simulink library "dspsigattribs"  (Simulink 6.0)
values from neighbouring files (symbols this model uses):
  D = D + B    [rebuffer_delay.m]
libraries: dspsigattribs x2, simulink x1, simulink3 x1
settings Model: RequirementInfo=9  CovMetricSettings=d  Creator=don  LastModifiedBy=mlongfri  ExtModeAutoUpdateStatusClock=off
settings Model: ForwardingTableString=|
  | ||__slOldName__||dspsigattribs/Contiguous
  | Copy||__slNewName__||dspobslib/Contiguous
  | Copy||__slOldName__||dspsigattribs/DSP Fixed-Point
  | Attributes||__slNewName__||dspobslib/DSP Fixed-Point
  | Attributes

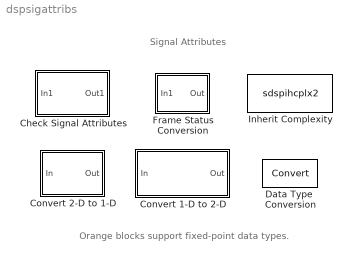
== system dspsigattribs ==
  note: Signal Attributes
  note: Orange blocks support fixed-point data types.
  Check Signal Attributes : Subsystem  mask(Check Signal Attributes){SigAttribCheckMethod=Does not match attributes exactly, Complexity=Ignore, Frame=Ignore, DimsCheckMethod=Ignore, Dimensions=1-D, DatatypeCheckMethod=Ignore, DatatypeGeneral=Boolean, DtypeFloatSpecific=Any floating-point, DtypeFixedSpecific=Any fixed-point, DtypeIntSpecific=Any integer, SampleMode=Ignore}
      mask prompts: SigAttribCheckMethod "Error when input:"; Frame "Frame status:"; DimsCheckMethod "Dimensionality:"; DatatypeCheckMethod "Data type:"; DatatypeGeneral "General data type:"; DtypeFloatSpecific "Specific floating-point:"; DtypeFixedSpecific "Specific fixed-point:"; DtypeIntSpecific "Specific integer:"; SampleMode "Sample mode:"
      mask help: Generate an error when the input signal does or does not match selected attributes exactly.
      settings: CopyFcn=dspfixptcopycallback
      mask Help: web(dspbhelp);
      mask StyleString: popup(Does not match attributes exactly|Matches attributes exactly),popup(Ignore|Real|Complex),popup(Ignore|Frame-based|Sample-based),popup(Ignore|Is...|Is not...),popup(1-D|2-D|Scalar (1-D or 2-D)|Vector (1-D or 2-D)|Vector (1-D or 2-D) or scalar|Row vector (2-D)|Row vector (2-D) or scalar|Column vector (2-D)|Column vector (2-D) or scalar|Full matrix (2-D)|Square matrix (2-D)),popup(Ignore|Is...|Is not...),popup(Boolean|Floating-point|Fixed-point|Integer),popup(Any floating-point|Double precision|Single precision),popup(Any fixed-point|Signed fixed-point|Unsigned fixed-point),popup(Any integer|Signed integer|Unsigned integer|int8|int16|int32|uint8|uint16|uint32),popup(Ignore|Discrete|Continuous)
      mask CallbackString: |||dspblkchksigattrbs||dspblkchksigattrbs|dspblkchksigattrbs|||dspblkchksigattrbs|
      mask Display: disp('Check Signal\n Attributes');
  Convert 1-D to 2-D : Subsystem  mask(Convert 1-D to 2-D){M=1, N=1, frameBasedOut=off}
      mask prompts: M "Number of output rows:"; N "Number of output columns:"; frameBasedOut "Frame-based output"
      mask help: Output a (2-D) matrix signal.
      mask init:
      | dspblkcnvrt1d2d;
      settings: CopyFcn=dspfixptcopycallback
      mask Help: web(dspbhelp);
      mask Display: disp('reshape(U,M,N)')
  Convert 2-D to 1-D : Subsystem
      settings: CopyFcn=dspfixptcopycallback
      mask Type: Convert 2-D to 1-D
      mask Description: Output a (1-D) vector signal.
      mask Help: web(dspbhelp);
      mask Display: disp('U( : )')
  Data Type  Conversion : DataTypeConversion  SaturateOnIntegerOverflow=on  RndMeth=Zero
      settings: CopyFcn=dspfixptcopycallback
  Frame Status Conversion : Subsystem  mask(Frame Status Conversion){growRefPort=off, outframe=Frame-based}
      mask prompts: growRefPort "Inherit output frame status from Ref input port"; outframe "Output signal:"
      mask help: Specify the frame status of the output signal.
      mask init:
      | [p, str] = dspblkfrmconv('init');
      settings: CopyFcn=dspfixptcopycallback
      mask Help: web(dspbhelp);
      mask StyleString: checkbox,popup(Frame-based|Sample-based)
      mask CallbackString: dspblkfrmconv|
      mask Display:
      | port_label(p.in1,   p.i1,  p.i1s);
      | port_label(p.in2,   p.i2,  p.i2s);
      | port_label(p.out, p.o1, p.o1s);
      | disp(str)
  Inherit Complexity : S-Function  FunctionName=sdspihcplx2
      settings: CopyFcn=dspfixptcopycallback
      mask Type: Inherit Complexity
      mask Description: Copy data from the Data input with the complexity of the reference signal. If the data is real and the reference is complex, an all zero imaginary part is created. If the data is complex and the reference is real, the imaginary part of the input is removed.
      mask Help: web(dspbhelp);
      mask Display:
      | text(.9,0.5,'Inherit\nComplexity','horiz','right');
      | port_label('input',1,'Data');
      | port_label('input',2,'Ref');

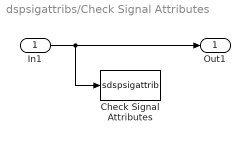
== system dspsigattribs/Check Signal Attributes ==
  In1 : Inport
  Check Signal Attributes : S-Function  FunctionName=sdspsigattrib  Parameters=SigAttribCheckMethod,Complexity,Frame,DimsCheckMethod,Dimensions,DatatypeCheckMethod,DatatypeGeneral,DtypeFloatSpecific,DtypeFixedSpecific,DtypeIntSpecific,SampleMode
  Out1 : Outport
  wires:
  In1/1 -> Out1/1, Check Signal Attributes/1

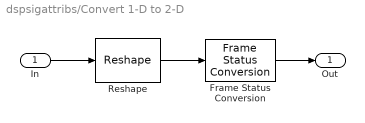
== system dspsigattribs/Convert 1-D to 2-D ==
  In : Inport
  Frame Status Conversion : dspsigattribs/Frame Status Conversion  growRefPort=off  outframe=Sample-based
  Reshape : simulink/Math Operations/Reshape  OutputDimensionality=Customize  OutputDimensions=[M,N]
  Out : Outport
  wires:
  Frame Status Conversion/1 -> Out/1
  In/1 -> Reshape/1
  Reshape/1 -> Frame Status Conversion/1

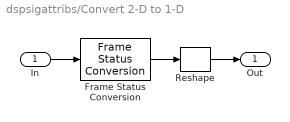
== system dspsigattribs/Convert 2-D to 1-D ==
  In : Inport
  Frame Status Conversion : dspsigattribs/Frame Status Conversion  growRefPort=off  outframe=Sample-based
  Reshape : simulink3/Signals & Systems/Reshape  OutputDimensionality=1-D array  OutputDimensions=[1,1]
  Out : Outport
  wires:
  Reshape/1 -> Out/1
  In/1 -> Frame Status Conversion/1
  Frame Status Conversion/1 -> Reshape/1

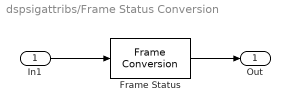
== system dspsigattribs/Frame Status Conversion ==
  In1 : Inport
  Frame Status : FrameConversion
  Out : Outport
  wires:
  In1/1 -> Frame Status/1
  Frame Status/1 -> Out/1
